simulink model "aero_atc"  (R2021b)
settings: Solver=ode45  StartTime=0.0  StopTime=10000  MaxStep=0.25  RelTol=1e-3  EnableMultiTasking=on
PreLoadFcn:
  | aero_atcgui;
InitFcn:
  | aero_init_atc
values from neighbouring files (symbols this model uses):
  AZ_Sep = get(findobj('Tag','AZ_Sep_edit'),'Value')    [aero_init_atc.m]
  BwPw = get(findobj('Tag','BW_PW_edit'),'Value')    [aero_init_atc.m]
  E = get(findobj('Tag','Antenna_E_edit'),'Value')    [aero_init_atc.m]
  EL_Sep = get(findobj('Tag','EL_Sep_edit'),'Value')    [aero_init_atc.m]
  Lambda = get(findobj('Tag','Wavelength_edit'),'Value')    [aero_init_atc.m]
  lambda_bp = [0.057    0.075   0.1     0.15    0.3]    [aero_init_atc.m]
  Loss = get(findobj('Tag','Losses_edit'),'Value')    [aero_init_atc.m]
  Noise = get(findobj('Tag','Noise_Factor_edit'),'Value')    [aero_init_atc.m]
  Pt = get(findobj('Tag','Trans_Power_edit'),'Value')    [aero_init_atc.m]
  rainfall = get(findobj('Style','radiobutton','Value',1),'UserData')    [aero_init_atc.m]
  rainfall_bp = [0        0.25    1       4       16]    [aero_init_atc.m]
  Rrange = get(findobj('Tag','RADAR_Range_edit'),'Value')    [aero_init_atc.m]
  Rres = get(findobj('Tag','Range_Res_edit'),'Value')    [aero_init_atc.m]
  sigma_table = [0.0      0.0     0.0     0.0     0.0;         7.5e-10  3.0e-10 8.5e-11 9.0e-12 9.0e-13;         6.5e-9   3.6e-9  7.0e-10 7.0e-11 7.0e-12;         7.5e-8   4.1e-8  6.8e-9  6.8e-10 6.8e-11;         7.0e-7   3.9e-7  8.0e-8  8.0e-9  8.0e-10]    [aero_init_atc.m]
  SNR = get(findobj('Tag','SNR_edit'),'Value')    [aero_init_atc.m]
  Temp = get(findobj('Tag','Working_Temp_edit'),'Value')    [aero_init_atc.m]
undefined symbols (not defined in the file or in its folder): Newton, Raphson
CloseFcn:
  | h = findobj('Type','figure','Name','Air Traffic RADAR Design Parameters');
  | if ~isempty(h)
  |     close(h);
  | end
Description:
  | Air traffic control demonstration
settings Model: RequirementInfo=9  FPTRunName=Active  Creator=The MathWorks, Inc.  LastModifiedBy=The MathWorks, Inc.
settings SolverCC: AlgebraicLoopSolver=TrustRegion
settings DataIOCC: MaxDataPoints=5000  SaveFormat=Array  SaveOutput=off  SignalLogging=off  SaveTime=off  ReturnWorkspaceOutputs=off
settings OptimizationCC: BlockReduction=off  BooleanDataType=off  ExpressionDepthLimit=2147483647  InitFltsAndDblsToZero=on  LifeSpan=inf
settings DebuggingCC: SaveWithParameterizedLinksMsg=none  CheckExecutionContextPreStartOutputMsg=on  SignalResolutionControl=TryResolveAllWithWarning  MultiTaskDSMMsg=warning  MultiTaskCondExecSysMsg=none  FcnCallInpInsideContextMsg=warning  AllowSymbolicDim=off  StateNameClashWarn=warning  SFUnexpectedBacktrackingDiag=warning  SFNoUnconditionalDefaultTransitionDiag=warning  SFExecutionAtInitializationDiag=none  SFMachineParentedDataDiag=warning  ArithmeticOperatorsInVariantConditions=warning
settings HardwareCC: ProdBitPerPointer=32  ProdBitPerSizeT=32  ProdBitPerPtrDiffT=32  ProdLargestAtomicFloat=None  ProdIntDivRoundTo=Undefined  ProdEndianess=Unspecified  ProdWordSize=32  ProdHWDeviceType=32-bit Generic
settings ModelReferenceCC: PropagateSignalLabelsOutOfModel=off
settings SFSimCC: SimUseLocalCustomCode=off  SimParseCustomCode=off  CustomCodeUndefinedFunction=UseInterfaceOnly
settings RTWCC: RTWUseLocalCustomCode=off
settings CodeAppCC: StateflowObjectComments=on
settings GRTTargetCC: TargetFcnLib=ansi_tfl_tmw.mat  TargetLangStandard=C89/C90 (ANSI)  CombineOutputUpdateFcns=off  GRTInterface=on
settings ConfigComp: CovMetricSettings=d  CovSaveCumulativeToWorkspaceVar=on  CovSaveSingleToWorkspaceVar=on  CovExternalEMLEnable=off  CovSFcnEnable=off

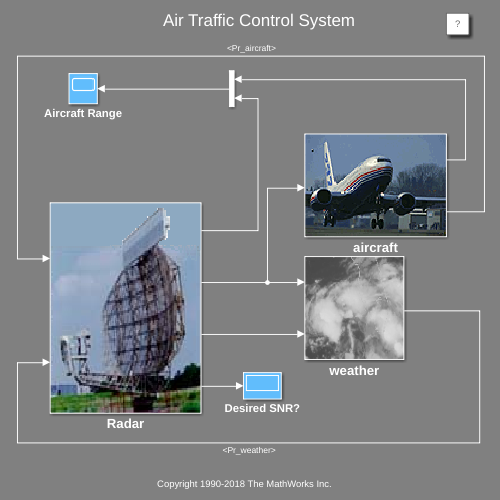
[thumbnail: Simulink's stored preview of the top-level diagram]
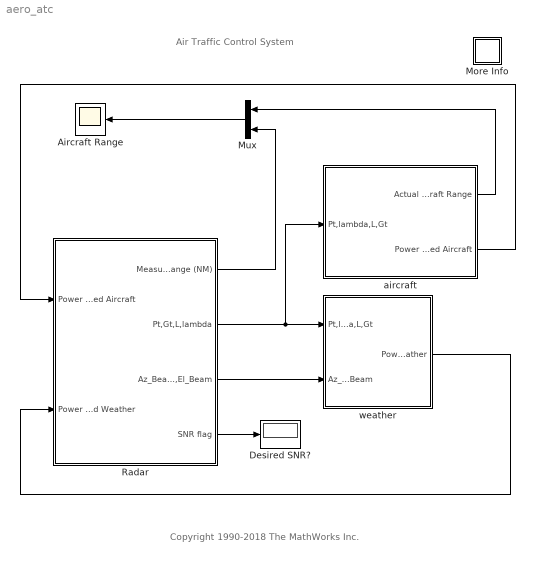
== system aero_atc ==
  note: Copyright 1990-2018 The MathWorks Inc.
  note: Air Traffic Control System
  Aircraft Range : Scope
  Desired SNR? : Display
  More Info : Subsystem
      settings: OpenFcn=showExample('simulink_aerospace/AirTrafficControlRadarDesignExample')
      mask Display: disp('?')
  Mux : Mux  Inputs=2
  Radar : Subsystem
      mask Display: image('$imagefile'); % Use "Edit Image" on toolstrip to change.
  aircraft : Subsystem
      mask Display: image('$imagefile'); % Use "Edit Image" on toolstrip to change.
  weather : Subsystem
      mask Display: image('$imagefile'); % Use "Edit Image" on toolstrip to change.
  wires:
  Radar/2(Pt,Gt,L,lambda) -> aircraft/1(Pt,lambda,L,Gt), weather/1(Pt,lambda,L,Gt)
  Radar/3(Az_Beam,El_Beam) -> weather/2(Az_Beam,El_Beam)
  weather/1(Power Returned Weather) -> Radar/2(Power Received Weather)
  aircraft/2(Power Returned Aircraft) -> Radar/1(Power Received Aircraft)
  Radar/1(Measured Aircraft Range (NM)) -> Mux/2
  aircraft/1(Actual Aircraft Range) -> Mux/1
  Mux/1 -> Aircraft Range/1
  Radar/4(SNR flag) -> Desired SNR?/1

== system aero_atc/More Info ==

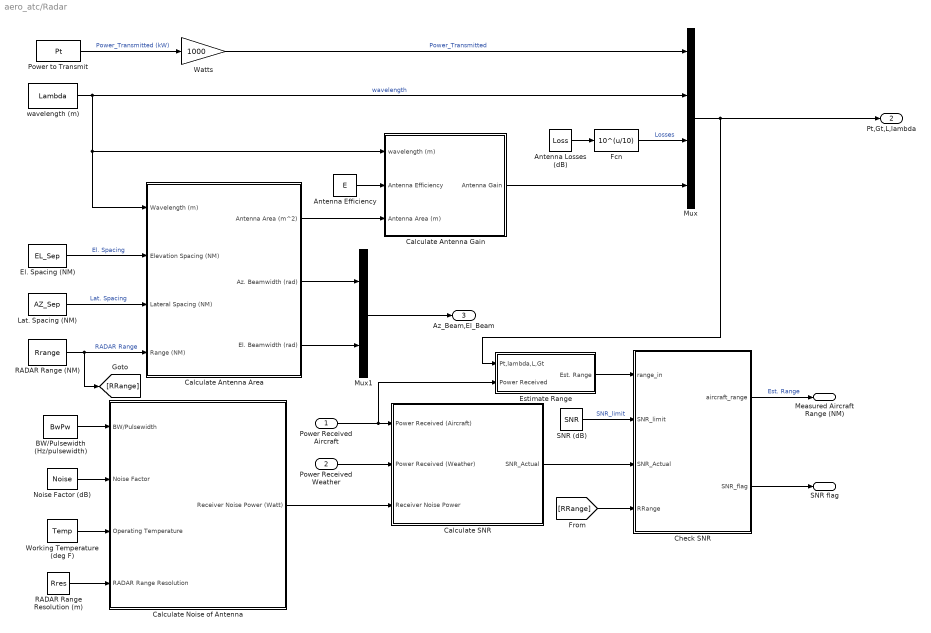
== system aero_atc/Radar ==
  Power Received Aircraft : Inport
  Power Received Weather : Inport  Port=2
  Antenna Efficiency : Constant  Value=E
  Antenna Losses (dB) : Constant  Value=Loss
  BW/Pulsewidth (Hz/pulsewidth) : Constant  Value=BwPw
  Calculate SNR : Subsystem
  Calculate Antenna Area : Subsystem
  Calculate Antenna Gain : Subsystem
  Calculate Noise of Antenna : Subsystem
  Check SNR : Stateflow chart  TreatAsAtomicUnit=on
  El. Spacing (NM) : Constant  Value=EL_Sep
  Estimate Range : Subsystem
  Fcn : Fcn  Expr=10^(u/10)
  Lat. Spacing (NM) : Constant  Value=AZ_Sep
  Mux : Mux
  Mux1 : Mux  Inputs=2
  Noise Factor (dB) : Constant  Value=Noise
  Power to Transmit : Constant  Value=Pt
  RADAR Range (NM) : Constant  Value=Rrange
  RADAR Range Resolution (m) : Constant  Value=Rres
  SNR (dB) : Constant  Value=SNR
  Watts : Gain  Gain=1000  SaturateOnIntegerOverflow=on  OutDataTypeStr=Inherit: Same as input  ParamDataTypeStr=Inherit: Same as input
  Working Temperature (deg F) : Constant  Value=Temp
  "wavelength (m) " : Constant  Value=Lambda
  Measured Aircraft Range (NM) : Outport  VectorParamsAs1DForOutWhenUnconnected=off
  Pt,Gt,L,lambda : Outport  Port=2  VectorParamsAs1DForOutWhenUnconnected=off
  Az_Beam,El_Beam : Outport  Port=3  VectorParamsAs1DForOutWhenUnconnected=off
  SNR flag : Outport  Port=4  VectorParamsAs1DForOutWhenUnconnected=off
  wires:
  Antenna Efficiency/1 -> Calculate Antenna Gain/2(Antenna Efficiency)
  Lat. Spacing (NM)/1 -> Calculate Antenna Area/3(Lateral Spacing (NM))  "Lat. Spacing"
  El. Spacing (NM)/1 -> Calculate Antenna Area/2(Elevation Spacing (NM))  "El. Spacing"
  "wavelength (m) "/1 -> Calculate Antenna Area/1(Wavelength (m)), Calculate Antenna Gain/1(wavelength (m)), Mux/2  "wavelength"
  Calculate Antenna Area/1(Antenna Area (m^2)) -> Calculate Antenna Gain/3(Antenna Area (m))
  RADAR Range (NM)/1 -> Calculate Antenna Area/4(Range (NM)), [RRange]  "RADAR Range"
  RADAR Range Resolution (m)/1 -> Calculate Noise of Antenna/4(RADAR Range Resolution)
  BW/Pulsewidth (Hz/pulsewidth)/1 -> Calculate Noise of Antenna/1(BW/Pulsewidth)
  Noise Factor (dB)/1 -> Calculate Noise of Antenna/2(Noise Factor)
  Working Temperature (deg F)/1 -> Calculate Noise of Antenna/3(Operating Temperature)
  Calculate Antenna Area/3("El. Beamwidth (rad) ") -> Mux1/2
  Calculate Antenna Area/2("Az. Beamwidth (rad) ") -> Mux1/1
  Mux1/1 -> Az_Beam,El_Beam/1
  Power Received Weather/1 -> Calculate SNR/2(Power Received (Weather))
  Power Received Aircraft/1 -> Calculate SNR/1(Power Received (Aircraft)), Estimate Range/2(Power Received)
  Calculate Noise of Antenna/1(Receiver Noise Power (Watt)) -> Calculate SNR/3(Receiver Noise Power)
  Mux/1 -> Pt,Gt,L,lambda/1, Estimate Range/1(Pt,lambda,L,Gt)
  Calculate Antenna Gain/1("Antenna Gain ") -> Mux/4
  Fcn/1 -> Mux/3  "Losses"
  Watts/1 -> Mux/1  "Power_Transmitted"
  Antenna Losses (dB)/1 -> Fcn/1
  Power to Transmit/1 -> Watts/1  "Power_Transmitted (kW)"
  Check SNR/1(aircraft_range) -> Measured Aircraft Range (NM)/1  "Est. Range"
  Estimate Range/1(Est. Range) -> Check SNR/1(range_in)
  SNR (dB)/1 -> Check SNR/2(SNR_limit)  "SNR_limit"
  Calculate SNR/1(SNR_Actual) -> Check SNR/3(SNR_Actual)
  [RRange] -> Check SNR/4(RRange)
  Check SNR/2(SNR_flag) -> SNR flag/1

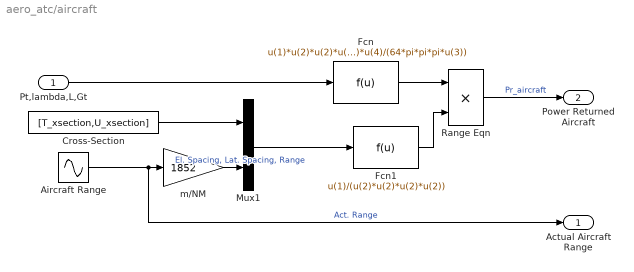
== system aero_atc/aircraft ==
  Pt,lambda,L,Gt : Inport
  Aircraft Range : Sin  Amplitude=25  Bias=35  Frequency=0.0025  SampleTime=0
  Cross-Section : FromWorkspace  VariableName=[T_xsection,U_xsection]  Interpolate=off  ZeroCross=off  OutputAfterFinalValue=Holding final value
  Fcn : Fcn  Expr=u(1)*u(2)*u(2)*u(4)*u(4)/(64*pi*pi*pi*u(3))
  Fcn1 : Fcn  Expr=u(1)/(u(2)*u(2)*u(2)*u(2))
  Mux1 : Mux  Inputs=2
  Range Eqn : Product  InputSameDT=on  RndMeth=Zero  SaturateOnIntegerOverflow=on  OutDataTypeStr=Inherit: Same as first input
  m/NM : Gain  Gain=1852  SaturateOnIntegerOverflow=on  OutDataTypeStr=Inherit: Same as input  ParamDataTypeStr=Inherit: Same as input
  Actual Aircraft Range : Outport  VectorParamsAs1DForOutWhenUnconnected=off
  Power Returned Aircraft : Outport  Port=2  VectorParamsAs1DForOutWhenUnconnected=off
  wires:
  Pt,lambda,L,Gt/1 -> Fcn/1
  Cross-Section/1 -> Mux1/1
  Mux1/1 -> Fcn1/1
  m/NM/1 -> Mux1/2  "El. Spacing, Lat. Spacing, Range"
  Fcn/1 -> Range Eqn/1
  Range Eqn/1 -> Power Returned Aircraft/1  "Pr_aircraft"
  Fcn1/1 -> Range Eqn/2
  Aircraft Range/1 -> Actual Aircraft Range/1, m/NM/1  "Act. Range"

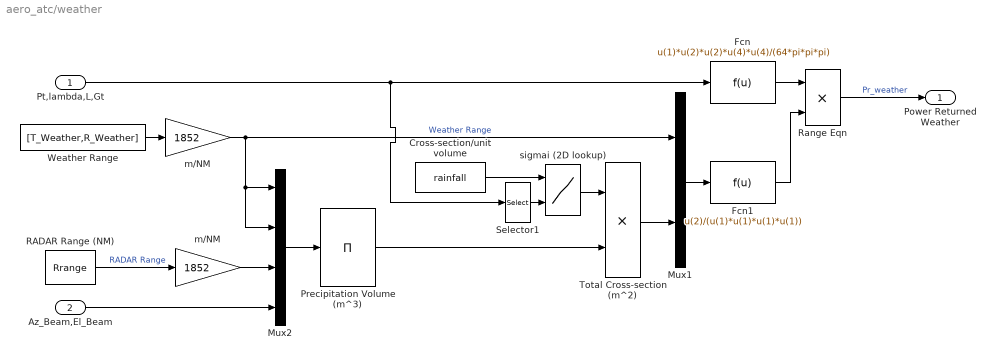
== system aero_atc/weather ==
  Pt,lambda,L,Gt : Inport
  Az_Beam,El_Beam : Inport  Port=2
  Cross-section/unit volume : Constant  Value=rainfall
  Fcn : Fcn  Expr=u(1)*u(2)*u(2)*u(4)*u(4)/(64*pi*pi*pi)
  Fcn1 : Fcn  Expr=u(2)/(u(1)*u(1)*u(1)*u(1))
  Mux1 : Mux  Inputs=2
  Mux2 : Mux
  Precipitation Volume (m^3) : Product  Inputs=*  InputSameDT=on  RndMeth=Zero  SaturateOnIntegerOverflow=on  OutDataTypeStr=Inherit: Same as first input
  RADAR Range (NM) : Constant  Value=Rrange
  Range Eqn : Product  InputSameDT=on  RndMeth=Zero  SaturateOnIntegerOverflow=on  OutDataTypeStr=Inherit: Same as first input
  Selector1 : Selector  InputPortWidth=4  IndexOptions=Index vector (dialog)  Indices=2  OutputSizes=1
  Total Cross-section (m^2) : Product  InputSameDT=on  RndMeth=Zero  SaturateOnIntegerOverflow=on  OutDataTypeStr=Inherit: Same as first input
  Weather Range : FromWorkspace  VariableName=[T_Weather,R_Weather]  Interpolate=off  ZeroCross=off  OutputAfterFinalValue=Holding final value
  m/NM : Gain  Gain=1852  SaturateOnIntegerOverflow=on  OutDataTypeStr=Inherit: Same as input  ParamDataTypeStr=Inherit: Same as input
  "m/NM " : Gain  Gain=1852  SaturateOnIntegerOverflow=on  OutDataTypeStr=Inherit: Same as input  ParamDataTypeStr=Inherit: Same as input
  sigmai (2D lookup) : Lookup_n-D  BreakpointsForDimension1=rainfall_bp  BreakpointsForDimension2=lambda_bp  Table=sigma_table  SaturateOnIntegerOverflow=on  InputSameDT=on
      settings: InputPortMap=u0,u1
  Power Returned Weather : Outport  VectorParamsAs1DForOutWhenUnconnected=off
  wires:
  Mux2/1 -> Precipitation Volume (m^3)/1
  m/NM/1 -> Mux2/3
  RADAR Range (NM)/1 -> m/NM/1  "RADAR Range"
  Az_Beam,El_Beam/1 -> Mux2/4
  "m/NM "/1 -> Mux1/1, Mux2/1, Mux2/2  "Weather Range"
  Mux1/1 -> Fcn1/1
  Weather Range/1 -> "m/NM "/1
  sigmai (2D lookup)/1 -> Total Cross-section (m^2)/1
  Pt,lambda,L,Gt/1 -> Selector1/1, Fcn/1
  Precipitation Volume (m^3)/1 -> Total Cross-section (m^2)/2
  Fcn1/1 -> Range Eqn/2
  Selector1/1 -> sigmai (2D lookup)/2
  Cross-section/unit volume/1 -> sigmai (2D lookup)/1
  Total Cross-section (m^2)/1 -> Mux1/2
  Fcn/1 -> Range Eqn/1
  Range Eqn/1 -> Power Returned Weather/1  "Pr_weather"

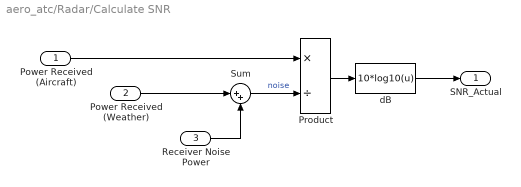
== system aero_atc/Radar/Calculate SNR ==
  Power Received (Aircraft) : Inport
  Power Received (Weather) : Inport  Port=2
  Receiver Noise Power : Inport  Port=3
  Product : Product  Inputs=*/  InputSameDT=on  RndMeth=Zero  SaturateOnIntegerOverflow=on  OutDataTypeStr=Inherit: Same as first input
  Sum : Sum  Inputs=|++  InputSameDT=on  SaturateOnIntegerOverflow=on  OutDataTypeStr=Inherit: Same as first input
  dB : Fcn  Expr=10*log10(u)
  SNR_Actual : Outport  VectorParamsAs1DForOutWhenUnconnected=off
  wires:
  Sum/1 -> Product/2  "noise"
  Power Received (Aircraft)/1 -> Product/1
  Power Received (Weather)/1 -> Sum/1
  Receiver Noise Power/1 -> Sum/2
  Product/1 -> dB/1
  dB/1 -> SNR_Actual/1

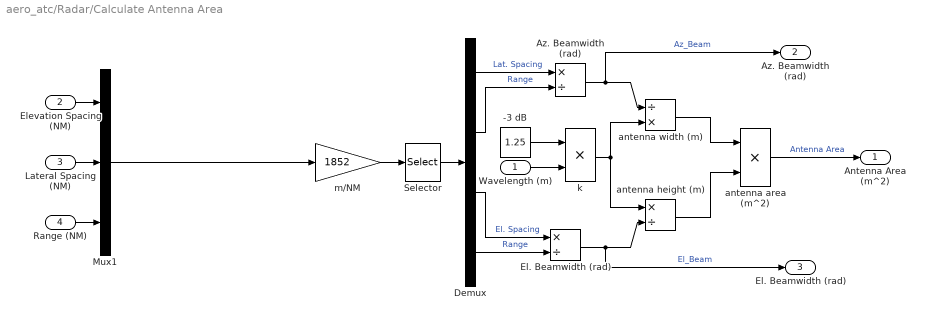
== system aero_atc/Radar/Calculate Antenna Area ==
  Wavelength (m) : Inport
  Elevation Spacing (NM) : Inport  Port=2
  Lateral Spacing (NM) : Inport  Port=3
  Range (NM) : Inport  Port=4
  "-3 dB  " : Constant  Value=1.25
  Az. Beamwidth (rad) : Product  Inputs=*/  InputSameDT=on  RndMeth=Zero  SaturateOnIntegerOverflow=on  OutDataTypeStr=Inherit: Same as first input
  Demux : Demux
      settings: DisplayOption=none
  El. Beamwidth (rad) : Product  Inputs=*/  InputSameDT=on  RndMeth=Zero  SaturateOnIntegerOverflow=on  OutDataTypeStr=Inherit: Same as first input
  Mux1 : Mux  Inputs=3
  Selector : Selector  InputPortWidth=3  IndexOptions=Index vector (dialog)  Indices=[1 3 2 3]  OutputSizes=1
  antenna area (m^2) : Product  InputSameDT=on  RndMeth=Zero  SaturateOnIntegerOverflow=on  OutDataTypeStr=Inherit: Same as first input
  antenna height (m) : Product  Inputs=*/  InputSameDT=on  RndMeth=Zero  SaturateOnIntegerOverflow=on  OutDataTypeStr=Inherit: Same as first input
  antenna width (m) : Product  Inputs=/*  InputSameDT=on  RndMeth=Zero  SaturateOnIntegerOverflow=on  OutDataTypeStr=Inherit: Same as first input
  k : Product  Inputs=**  InputSameDT=on  RndMeth=Zero  SaturateOnIntegerOverflow=on  OutDataTypeStr=Inherit: Same as first input
  m/NM : Gain  Gain=1852  SaturateOnIntegerOverflow=on  OutDataTypeStr=Inherit: Same as input  ParamDataTypeStr=Inherit: Same as input
  Antenna Area (m^2) : Outport  VectorParamsAs1DForOutWhenUnconnected=off
  "Az. Beamwidth (rad) " : Outport  Port=2  VectorParamsAs1DForOutWhenUnconnected=off
  "El. Beamwidth (rad) " : Outport  Port=3  VectorParamsAs1DForOutWhenUnconnected=off
  wires:
  m/NM/1 -> Selector/1
  Selector/1 -> Demux/1
  Demux/1 -> Az. Beamwidth (rad)/1  "Lat. Spacing"
  Demux/2 -> Az. Beamwidth (rad)/2  "Range"
  Demux/3 -> El. Beamwidth (rad)/1  "El. Spacing"
  Demux/4 -> El. Beamwidth (rad)/2  "Range"
  Wavelength (m)/1 -> k/2
  "-3 dB  "/1 -> k/1
  k/1 -> antenna height (m)/1, antenna width (m)/2
  Az. Beamwidth (rad)/1 -> antenna width (m)/1, "Az. Beamwidth (rad) "/1  "Az_Beam"
  antenna width (m)/1 -> antenna area (m^2)/1
  antenna height (m)/1 -> antenna area (m^2)/2
  antenna area (m^2)/1 -> Antenna Area (m^2)/1  "Antenna Area"
  El. Beamwidth (rad)/1 -> antenna height (m)/2, "El. Beamwidth (rad) "/1  "El_Beam"
  Mux1/1 -> m/NM/1
  Elevation Spacing (NM)/1 -> Mux1/1
  Lateral Spacing (NM)/1 -> Mux1/2
  Range (NM)/1 -> Mux1/3

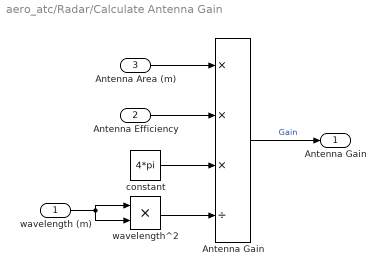
== system aero_atc/Radar/Calculate Antenna Gain ==
  wavelength (m) : Inport
  Antenna Efficiency : Inport  Port=2
  Antenna Area (m) : Inport  Port=3
  Antenna Gain : Product  Inputs=***/  InputSameDT=on  RndMeth=Zero  SaturateOnIntegerOverflow=on  OutDataTypeStr=Inherit: Same as first input
  constant : Constant  Value=4*pi
  wavelength^2 : Product  InputSameDT=on  RndMeth=Zero  SaturateOnIntegerOverflow=on  OutDataTypeStr=Inherit: Same as first input
  "Antenna Gain " : Outport  VectorParamsAs1DForOutWhenUnconnected=off
  wires:
  Antenna Efficiency/1 -> Antenna Gain/2
  constant/1 -> Antenna Gain/3
  wavelength^2/1 -> Antenna Gain/4
  Antenna Area (m)/1 -> Antenna Gain/1
  Antenna Gain/1 -> "Antenna Gain "/1  "Gain"
  wavelength (m)/1 -> wavelength^2/2, wavelength^2/1

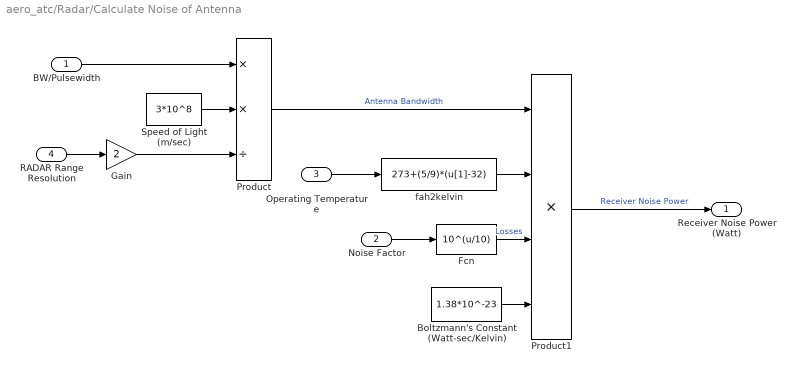
== system aero_atc/Radar/Calculate Noise of Antenna ==
  BW/Pulsewidth : Inport
  Noise Factor : Inport  Port=2
  Operating Temperature : Inport  Port=3
  RADAR Range Resolution : Inport  Port=4
  Boltzmann's Constant (Watt-sec/Kelvin) : Constant  Value=1.38*10^-23
  Fcn : Fcn  Expr=10^(u/10)
  Gain : Gain  Gain=2  SaturateOnIntegerOverflow=on  OutDataTypeStr=Inherit: Same as input  ParamDataTypeStr=Inherit: Same as input
  Product : Product  Inputs=**/  InputSameDT=on  RndMeth=Zero  SaturateOnIntegerOverflow=on  OutDataTypeStr=Inherit: Same as first input
  Product1 : Product  Inputs=4  InputSameDT=on  RndMeth=Zero  SaturateOnIntegerOverflow=on  OutDataTypeStr=Inherit: Same as first input
  Speed of Light (m/sec) : Constant  Value=3*10^8
  fah2kelvin : Fcn  Expr=273+(5/9)*(u[1]-32)
  Receiver Noise Power (Watt) : Outport  VectorParamsAs1DForOutWhenUnconnected=off
  wires:
  Speed of Light (m/sec)/1 -> Product/2
  Gain/1 -> Product/3
  BW/Pulsewidth/1 -> Product/1
  RADAR Range Resolution/1 -> Gain/1
  Product/1 -> Product1/1  "Antenna Bandwidth"
  fah2kelvin/1 -> Product1/2
  Boltzmann's Constant (Watt-sec/Kelvin)/1 -> Product1/4
  Product1/1 -> Receiver Noise Power (Watt)/1  "Receiver Noise Power"
  Noise Factor/1 -> Fcn/1
  Fcn/1 -> Product1/3  "Losses"
  Operating Temperature/1 -> fah2kelvin/1

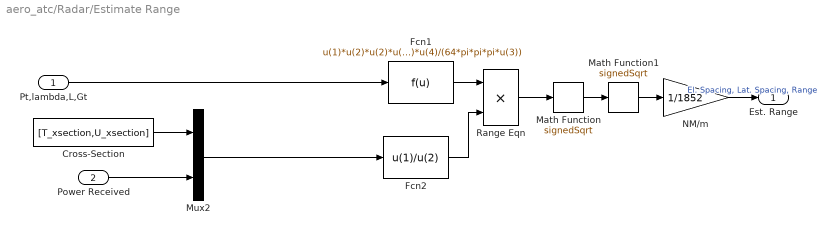
== system aero_atc/Radar/Estimate Range ==
  Pt,lambda,L,Gt : Inport
  Power Received : Inport  Port=2
  Cross-Section : FromWorkspace  VariableName=[T_xsection,U_xsection]  ZeroCross=off
  Fcn1 : Fcn  Expr=u(1)*u(2)*u(2)*u(4)*u(4)/(64*pi*pi*pi*u(3))
  Fcn2 : Fcn  Expr=u(1)/u(2)
  Math Function : Sqrt  Operator=signedSqrt  AlgorithmType=Newton-Raphson  SaturateOnIntegerOverflow=on
  Math Function1 : Sqrt  Operator=signedSqrt  AlgorithmType=Newton-Raphson  SaturateOnIntegerOverflow=on
  Mux2 : Mux  Inputs=2
  NM/m : Gain  Gain=1/1852  SaturateOnIntegerOverflow=on  OutDataTypeStr=Inherit: Same as input  ParamDataTypeStr=Inherit: Same as input
  Range Eqn : Product  InputSameDT=on  RndMeth=Zero  SaturateOnIntegerOverflow=on  OutDataTypeStr=Inherit: Same as first input
  Est. Range : Outport  VectorParamsAs1DForOutWhenUnconnected=off
  wires:
  Pt,lambda,L,Gt/1 -> Fcn1/1
  Fcn1/1 -> Range Eqn/1
  Fcn2/1 -> Range Eqn/2
  Range Eqn/1 -> Math Function/1
  Math Function/1 -> Math Function1/1
  Math Function1/1 -> NM/m/1
  NM/m/1 -> Est. Range/1  "El. Spacing, Lat. Spacing, Range"
  Cross-Section/1 -> Mux2/1
  Power Received/1 -> Mux2/2
  Mux2/1 -> Fcn2/1

== stateflow chart aero_atc/Radar/Check SNR ==
  settings: updateMethod=CONTINUOUS
  state Visibility [parallel]
    settings: executionOrder=1
    state detect
      during: aircraft_range = range_in;
    state no_detect
      during: aircraft_range =0;
    (default) -> (junction 17)
    (junction 17) -> no_detect [order 1] : [(SNR_Actual <= 6) || (range_in > RRange)]
        | { aircraft_range =0;}
    (junction 17) -> detect [order 2] : %(SNR_Actual > 6) && (range_in <= RRange)
        | { aircraft_range = range_in;}
    no_detect -> detect : [(SNR_Actual > 6) && (range_in <= RRange)]
        | { aircraft_range = range_in;}
    detect -> no_detect : [(SNR_Actual <= 6) || (range_in > RRange)]
        | { aircraft_range = 0;}
  state SNR [parallel]
    settings: executionOrder=2
    state Less_than
    state Equal_to_or_Greater_than
    (default) -> (junction 18)
    (junction 18) -> Less_than [order 2] : %SNR_Actual < SNR_limit
        | {SNR_flag = 0;}
    (junction 18) -> Equal_to_or_Greater_than [order 1] : [SNR_Actual >= SNR_limit]{SNR_flag = 1;}
    Less_than -> Equal_to_or_Greater_than : [SNR_Actual >= SNR_limit]{SNR_flag = 1;}
    Equal_to_or_Greater_than -> Less_than : [SNR_Actual < SNR_limit]{SNR_flag = 0;}
  data: range_in input double size=1; SNR_limit input double size=1; SNR_Actual input double size=1; aircraft_range output double size=1 =0; RRange input double size=1; SNR_flag output double size=1
